simulink subsystem "DropBits"  (R2024a)
settings: Solver=VariableStepAuto  StartTime=0.0  StopTime=10.0  RelTol=1e-3
libraries: hdlsllib x2
settings Model: Creator=versal  LastModifiedBy=versal

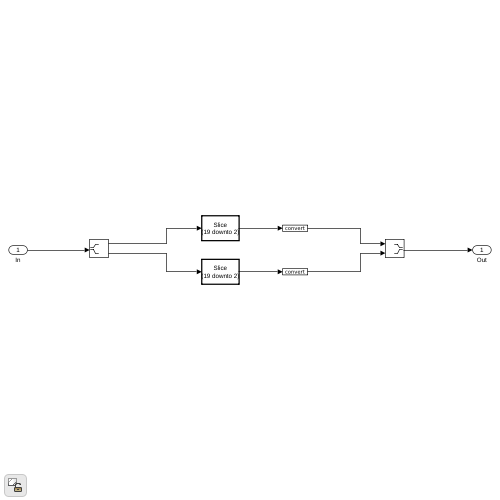
[thumbnail: Simulink's stored preview of the top-level diagram]
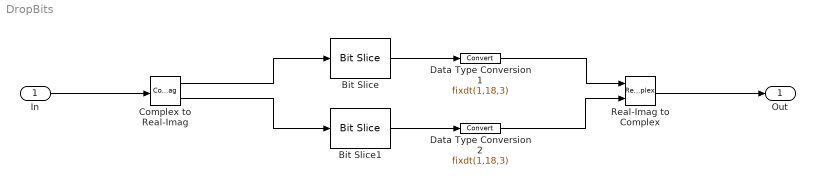
== system DropBits ==
  In : Inport
  Bit Slice : hdlsllib/Logic and Bit Operations/Bit Slice  lidx=19  ridx=2
  Bit Slice1 : hdlsllib/Logic and Bit Operations/Bit Slice  lidx=19  ridx=2
  Complex to Real-Imag : ComplexToRealImag
  Data Type Conversion1 : DataTypeConversion  OutDataTypeStr=fixdt(1,18,3)  SaturateOnIntegerOverflow=off  RndMeth=Floor
  Data Type Conversion2 : DataTypeConversion  OutDataTypeStr=fixdt(1,18,3)  SaturateOnIntegerOverflow=off  RndMeth=Floor
  Real-Imag to Complex : RealImagToComplex
  Out : Outport
  wires:
  Bit Slice/1 -> Data Type Conversion1/1
  Complex to Real-Imag/1 -> Bit Slice/1
  In/1 -> Complex to Real-Imag/1
  Data Type Conversion1/1 -> Real-Imag to Complex/1
  Real-Imag to Complex/1 -> Out/1
  Bit Slice1/1 -> Data Type Conversion2/1
  Complex to Real-Imag/2 -> Bit Slice1/1
  Data Type Conversion2/1 -> Real-Imag to Complex/2
